simulink model "model1"  (Simulink 7.7)
settings: Solver=VariableStepDiscrete  StartTime=0.0  StopTime=10.0  RelTol=1e-3
values from neighbouring files (symbols this model uses):
  A = A1'    [dyskretny.m]    (also in przebieg.m; zmiennestanu.m)
  C = B1'    [dyskretny.m]    (also in przebieg.m; zmiennestanu.m)
  K = acker(A, B,[z1, z2, z3])    [przebieg.m]    (also in zad4a.m = acker(A, B,[z, z, z]); zad4b.m = acker(A, B,[z, 0.0001, 0.0001]); zad4c.m = acker(A, B,[z, conj(z), 0.0001]); zmiennestanu.m = acker(A, B,[0.004600000000000 - 0.000400000000000i, conj(0.0)
  T_s = 0.25    [dyskretny.m]    (also in projekt.m; przebieg.m; zmiennestanu.m)
libraries: simulink x3
settings Model: Creator=Andones  LastModifiedBy=qiubix

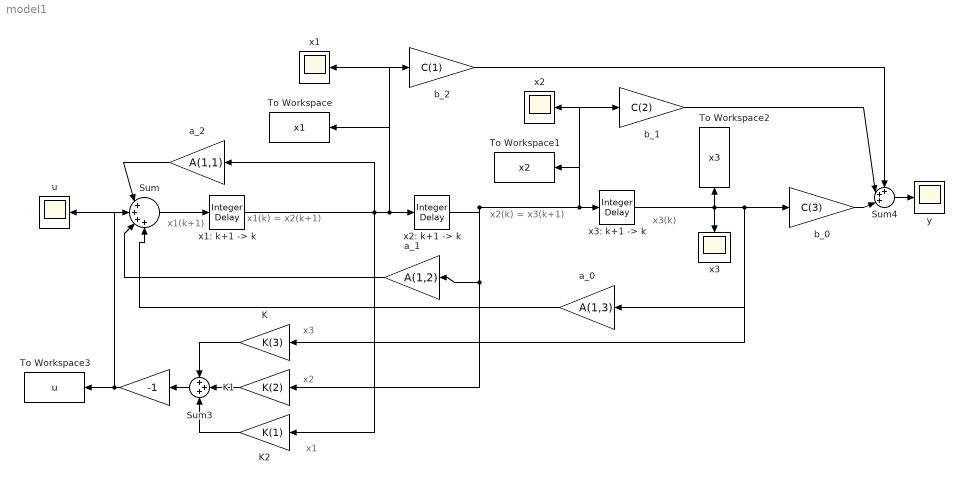
== system model1 ==
  note: x1(k+1)
  note: x3(k)
  note: x2
  note: x3
  note: x1
  note: x1(k) = x2(k+1)
  note: x2(k) = x3(k+1)
  " " : Gain  Gain=-1  SampleTime=T_s
  " x3: k+1 -> k" : simulink/Discrete/Integer Delay  NumDelays=1  vinit=1  samptime=T_s
  K : Gain  Gain=K(3)  SampleTime=T_s
  K1 : Gain  Gain=K(2)  SampleTime=T_s
  K2 : Gain  Gain=K(1)  SampleTime=T_s
  Sum : Sum  Inputs=|++++
  Sum3 : Sum  Inputs=+++
  Sum4 : Sum  Inputs=+++|
  To Workspace : ToWorkspace  VariableName=x1  SampleTime=T_s  SaveFormat=Array
  To Workspace1 : ToWorkspace  VariableName=x2  SampleTime=T_s  SaveFormat=Array
  To Workspace2 : ToWorkspace  VariableName=x3  SampleTime=T_s  SaveFormat=Array
  To Workspace3 : ToWorkspace  VariableName=u  SampleTime=T_s  SaveFormat=Array
  a_0 : Gain  Gain=A(1,3)
  a_1 : Gain  Gain=A(1,2)
  a_2 : Gain  Gain=A(1,1)
  b_0 : Gain  Gain=C(3)
  b_1 : Gain  Gain=C(2)
  b_2 : Gain  Gain=C(1)
  u : Scope
  x1 : Scope
      settings: SaveName=ScopeData2
  "x1: k+1 -> k " : simulink/Discrete/Integer Delay  NumDelays=1  vinit=-1  samptime=T_s
  x2 : Scope
      settings: SaveName=ScopeData3
  "x2: k+1 -> k" : simulink/Discrete/Integer Delay  NumDelays=1  vinit=-1  samptime=T_s
  x3 : Scope
      settings: SaveName=ScopeData4
  y : Scope
  wires:
  Sum/1 -> "x1: k+1 -> k "/1
  K1/1 -> Sum3/2
  K/1 -> Sum3/1
  K2/1 -> Sum3/3
  Sum3/1 -> " "/1
  Sum4/1 -> y/1
  b_0/1 -> Sum4/3
  b_1/1 -> Sum4/2
  b_2/1 -> Sum4/1
  "x1: k+1 -> k "/1 -> "x2: k+1 -> k"/1, b_2/1, x1/1, To Workspace/1, a_2/1, K2/1
  "x2: k+1 -> k"/1 -> " x3: k+1 -> k"/1, x2/1, b_1/1, To Workspace1/1, a_1/1, K1/1
  a_2/1 -> Sum/1
  a_0/1 -> Sum/4
  a_1/1 -> Sum/3
  " "/1 -> To Workspace3/1, Sum/2, u/1
  " x3: k+1 -> k"/1 -> To Workspace2/1, x3/1, b_0/1, a_0/1, K/1
